simulink model "DCMotor"  (R2014a)
settings: Solver=ode23t  StartTime=0.0  StopTime=15
libraries: fl_lib x13, nesl_utility x6, powerlib x1
settings Model: Creator=nicsi  LastModifiedBy=nicsi
settings SolverCC: SolverResetMethod=Robust  PositivePriorityOrder=on
settings DebuggingCC: AlgebraicLoopMsg=error  SolverPrmCheckMsg=none

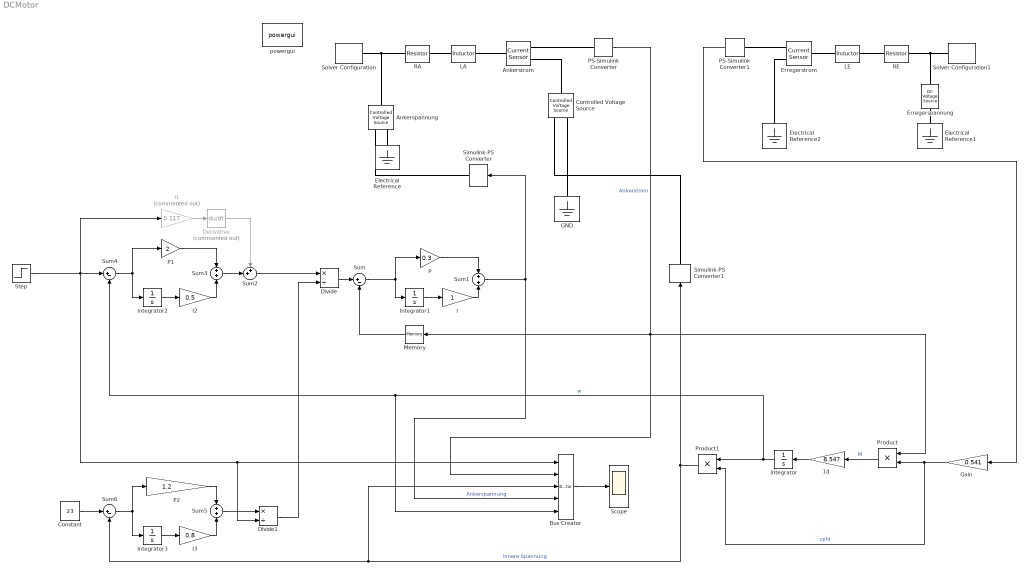
== system DCMotor ==
  "1/J " : Gain  Gain=8.547
  Ankerspannung : fl_lib/Electrical/Electrical Sources/Controlled Voltage Source
  Ankerstrom : fl_lib/Electrical/Electrical Sensors/Current Sensor
  Bus Creator : BusCreator  Inputs=5
  Constant : Constant  Value=23
  Controlled Voltage Source : fl_lib/Electrical/Electrical Sources/Controlled Voltage Source
  Derivative : Derivative  Commented=on
  Divide : Product  Inputs=*/
  Divide1 : Product  Inputs=*/
  Electrical Reference : fl_lib/Electrical/Electrical Elements/Electrical Reference
  Electrical Reference1 : fl_lib/Electrical/Electrical Elements/Electrical Reference
  Electrical Reference2 : fl_lib/Electrical/Electrical Elements/Electrical Reference
  Erregerspannung : fl_lib/Electrical/Electrical Sources/DC Voltage Source  v0=220 V
  "Erregerstrom " : fl_lib/Electrical/Electrical Sensors/Current Sensor
  GND : fl_lib/Electrical/Electrical Elements/Electrical Reference
  Gain : Gain  Gain=0.541
  I : Gain
  I1 : Gain  Commented=on  Gain=0.117
  I2 : Gain  Gain=0.5
  I3 : Gain  Gain=0.8
  Integrator{,1..3} (4 alike) : Integrator
  LA : fl_lib/Electrical/Electrical Elements/Inductor  l=26 mH  r=0 Ohm  g=1e-9 1/Ohm  i_specify=off  i_priority=High  i=0 A  v_specify=off  v_priority=High  v=0 V  i_L_specify=off  i_L_priority=High  i_L=0 A
  LE : fl_lib/Electrical/Electrical Elements/Inductor  l=20 H  r=0 Ohm  g=1e-9 1/Ohm  i_specify=off  i_priority=High  i=0 A  v_specify=off  v_priority=High  v=0 V  i_L_specify=off  i_L_priority=High  i_L=0 A
  Memory : Memory
  P : Gain  Gain=0.3
  P1 : Gain  Gain=2
  P2 : Gain  Gain=1.2
  PS-Simulink Converter : nesl_utility/PS-Simulink Converter  PhysicalDomain=network_engine_domain  SubClassName=ps_output  LeftPortType=input  RightPortType=output  PseudoPeriodic=off  Frequencies=[]  Unit=1  AffineConversion=off
  PS-Simulink Converter1 : nesl_utility/PS-Simulink Converter  PhysicalDomain=network_engine_domain  SubClassName=ps_output  LeftPortType=input  RightPortType=output  PseudoPeriodic=off  Frequencies=[]  Unit=1  AffineConversion=off
  Product : Product
  Product1 : Product
  "RA " : fl_lib/Electrical/Electrical Elements/Resistor  R=2.6 Ohm  i_specify=off  i_priority=High  i=0 A  v_specify=off  v_priority=High  v=0 V
  RE : fl_lib/Electrical/Electrical Elements/Resistor  R=100 Ohm  i_specify=off  i_priority=High  i=0 A  v_specify=off  v_priority=High  v=0 V
  Scope : Scope
      settings: ShowLegends=on  TimeRange=2  YMin=-7.5e+12  YMax=3.75e+13
  Simulink-PS Converter : nesl_utility/Simulink-PS Converter  PhysicalDomain=network_engine_domain  SubClassName=ps_input  LeftPortType=input  RightPortType=output  PseudoPeriodic=off  Frequencies=[]  NoiseDistribution=none  NoiseParameters=[]  Unit=1  AffineConversion=off  InputFiltering=off  SimscapeFilterOrder=1  InputFilterTimeConstant=0.001  UdotUserProvided=1
  Simulink-PS Converter1 : nesl_utility/Simulink-PS Converter  PhysicalDomain=network_engine_domain  SubClassName=ps_input  LeftPortType=input  RightPortType=output  PseudoPeriodic=off  Frequencies=[]  NoiseDistribution=none  NoiseParameters=[]  Unit=1  AffineConversion=off  InputFiltering=off  SimscapeFilterOrder=1  InputFilterTimeConstant=0.001  UdotUserProvided=1
  Solver Configuration : nesl_utility/Solver Configuration  PhysicalDomain=network_engine_domain  SubClassName=solver  LeftPortType=input  RightPortType=generic  Accelerate=off  Tones=[]  Harmonics=[]  SimulateNoise=off  Profile=off  UseLocalSampling=off  EnableSwitchedLinearOptims=on  FrequencyDomain=off  UseCCode=off  RelTol=0.001  AbsTol=1e-06  MinStep=1e-09  ToWorkspace=off  DoDC=on  ResidualTolerance=1e-09  UseLocalSolver=off  LocalSolverChoice=NE_BACKWARD_EULER_ADVANCER  LocalSolverSampleTime=0.001  DoFixedCost=off  MaxNonlinIter=3  MaxModeIter=2  LinearAlgebra=Sparse  DelaysMemoryBudget=1024  AutomaticFiltering=on  FilteringTimeConstant=0.001
  Solver Configuration1 : nesl_utility/Solver Configuration  PhysicalDomain=network_engine_domain  SubClassName=solver  LeftPortType=input  RightPortType=generic  Accelerate=off  Tones=[]  Harmonics=[]  SimulateNoise=off  Profile=off  UseLocalSampling=off  EnableSwitchedLinearOptims=on  FrequencyDomain=off  UseCCode=off  RelTol=0.001  AbsTol=1e-06  MinStep=1e-09  ToWorkspace=off  DoDC=on  ResidualTolerance=1e-09  UseLocalSolver=off  LocalSolverChoice=NE_BACKWARD_EULER_ADVANCER  LocalSolverSampleTime=0.001  DoFixedCost=off  MaxNonlinIter=3  MaxModeIter=2  LinearAlgebra=Sparse  DelaysMemoryBudget=1024  AutomaticFiltering=on  FilteringTimeConstant=0.001
  Step : Step  After=20  SampleTime=0
  Sum : Sum  Inputs=|+-
  Sum1 : Sum  Inputs=+|+
  Sum2 : Sum  Inputs=++|
  Sum3 : Sum  Inputs=+|+
  Sum4 : Sum  Inputs=|+-
  Sum5 : Sum  Inputs=+|+
  Sum6 : Sum  Inputs=|+-
  powergui : powerlib/powergui  Priority=1  SimulationMode=Continuous  SolverType=Tustin  SampleTime=50e-6  frequency=60  SPID=off  DisableSnubberDevices=off  DisableRonSwitches=off  DisableVfSwitches=off  SwTol=0  Interpol=off  DisplayEquations=off  Ts=0  methode=off  frequencyindice=60  Pbase=100e6  ErrMax=1e-4  Iterations=50  UnitsV=kV  UnitsW=MW  FunctionMessages=off  echomessages=off  HookPort=off  EnableUseOfTLC=off  x0status=blocks  RestoreLinks=warning  ResistiveCurrentMeasurement=off  Frange=[0:2:500]  Ylog=off  Xlog=on  ShowGrid=off  save=off  variable=ZData  structure=0  ZoomFFT=off  StartTime=0.0  cycles=1  DisplayStyle=1  fundamental=60  FreqAxis=off  MaxFrequency=1000  frequencyindicesteady=1  RmsSteady=1  display=off
  wires:
  PS-Simulink Converter/1 -> Bus Creator/2, Product/1, Memory/1  "Ankerstrom"
  Product/1 -> "1/J "/1  "M"
  "1/J "/1 -> Integrator/1
  Integrator/1 -> Product1/1, Sum4/2, Bus Creator/5  "w"
  Product1/1 -> Bus Creator/3, Sum6/2, Simulink-PS Converter1/1  "innere Spannung"
  Gain/1 -> Product/2, Product1/2  "cphi"
  Sum/1 -> Integrator1/1, P/1
  Integrator1/1 -> I/1
  I/1 -> Sum1/2
  P/1 -> Sum1/1
  PS-Simulink Converter1/1 -> Gain/1
  Bus Creator/1 -> Scope/1
  Sum1/1 -> Simulink-PS Converter/1, Bus Creator/4  "Ankerspannung"
  Divide/1 -> Sum/1
  Step/1 -> I1/1, Divide1/2, Bus Creator/1, Sum4/1
  Derivative/1 -> Sum2/1
  Sum2/1 -> Divide/1
  I1/1 -> Derivative/1
  Integrator2/1 -> I2/1
  I2/1 -> Sum3/2
  P1/1 -> Sum3/1
  Sum3/1 -> Sum2/2
  Sum4/1 -> P1/1, Integrator2/1
  Memory/1 -> Sum/2
  Integrator3/1 -> I3/1
  I3/1 -> Sum5/2
  P2/1 -> Sum5/1
  Sum6/1 -> P2/1, Integrator3/1
  Sum5/1 -> Divide1/1
  Divide1/1 -> Divide/2
  Constant/1 -> Sum6/1
  connections:
  Ankerspannung/LConn1 -- Solver Configuration/RConn1 -- "RA "/LConn1
  Simulink-PS Converter/RConn1 -- Ankerspannung/RConn1
  Ankerspannung/RConn2 -- Electrical Reference/LConn1
  "RA "/RConn1 -- LA/LConn1
  LA/RConn1 -- Ankerstrom/LConn1
  Ankerstrom/RConn1 -- PS-Simulink Converter/LConn1
  Electrical Reference1/LConn1 -- Erregerspannung/RConn1
  RE/LConn1 -- Solver Configuration1/RConn1 -- Erregerspannung/LConn1
  RE/RConn1 -- LE/LConn1
  "Erregerstrom "/LConn1 -- LE/RConn1
  "Erregerstrom "/RConn1 -- PS-Simulink Converter1/LConn1
  "Erregerstrom "/RConn2 -- Electrical Reference2/LConn1
  Controlled Voltage Source/LConn1 -- Ankerstrom/RConn2
  Controlled Voltage Source/RConn2 -- GND/LConn1
  Simulink-PS Converter1/RConn1 -- Controlled Voltage Source/RConn1
